simulink model "mechanikai"  (R2023b)
settings: Solver=ode45  StartTime=0.0  StopTime=1000  MaxStep=0.1  RelTol=1e-3
values from neighbouring files (symbols this model uses):
  b = 10    [lengorendszer.m]
  k = 15    [lengorendszer.m]
  m = 100    [lengorendszer.m]
libraries: simulink x1
settings Model: Creator=Meli  LastModifiedBy=puska
settings DebuggingCC: UnconnectedInputMsg=warning  UnconnectedOutputMsg=warning  UnconnectedLineMsg=warning
settings ModelReferenceCC: EnableRefExpFcnMdlSchedulingChecks=on
settings RTWCC: DLArmComputeVersion=19.05

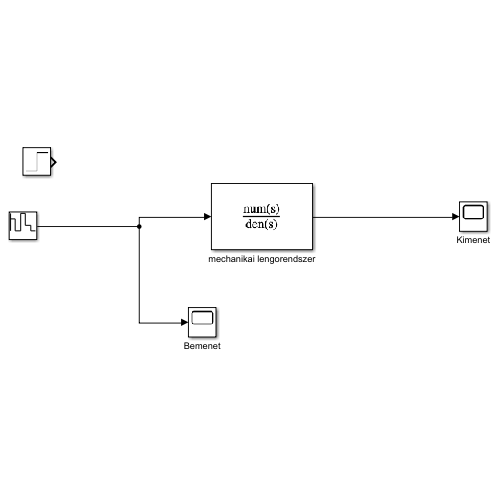
[thumbnail: Simulink's stored preview of the top-level diagram]
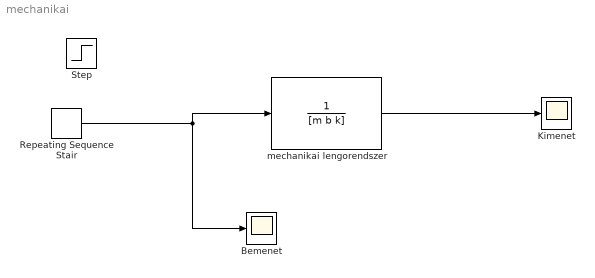
== system mechanikai ==
  Bemenet : Scope
  Kimenet : Scope
  Repeating Sequence Stair : simulink/Sources/Repeating Sequence Stair  OutValues=[3 1 4 2 1].'  tsamp=100  OutMin=[]  OutMax=[]  OutDataTypeStr=double  OutputDataTypeScalingMode=double  OutDataType=fixdt(0,8)  ConRadixGroup=Best Precision: Vector-wise  OutScaling=2^-12
  Step : Step  SampleTime=0
  mechanikai lengorendszer : TransferFcn  Numerator=1  Denominator=[m b k]
  wires:
  mechanikai lengorendszer/1 -> Kimenet/1
  Repeating Sequence Stair/1 -> mechanikai lengorendszer/1, Bemenet/1
